simulink model "highwind"  (Simulink 8.0)
settings: Solver=ode45  StartTime=0.0  StopTime=300.0  RelTol=1e-3
undefined symbols (not defined in the file or in its folder): c1, c2, c3, c4, c5, c6, ctrlpara, Jg, Jr, K, Kt, R, ro_air, xishu
libraries: simulink_need_slupdate x1, wt_blockset_v3 x1
settings Model: Creator=acer  LastModifiedBy=Administrator
settings DataIOCC: SignalLoggingSaveFormat=ModelDataLogs
settings DebuggingCC: FcnCallInpInsideContextMsg=UseLocalSettings  StrictBusMsg=Warning
settings GRTTargetCC: CombineOutputUpdateFcns=off  GRTInterface=on

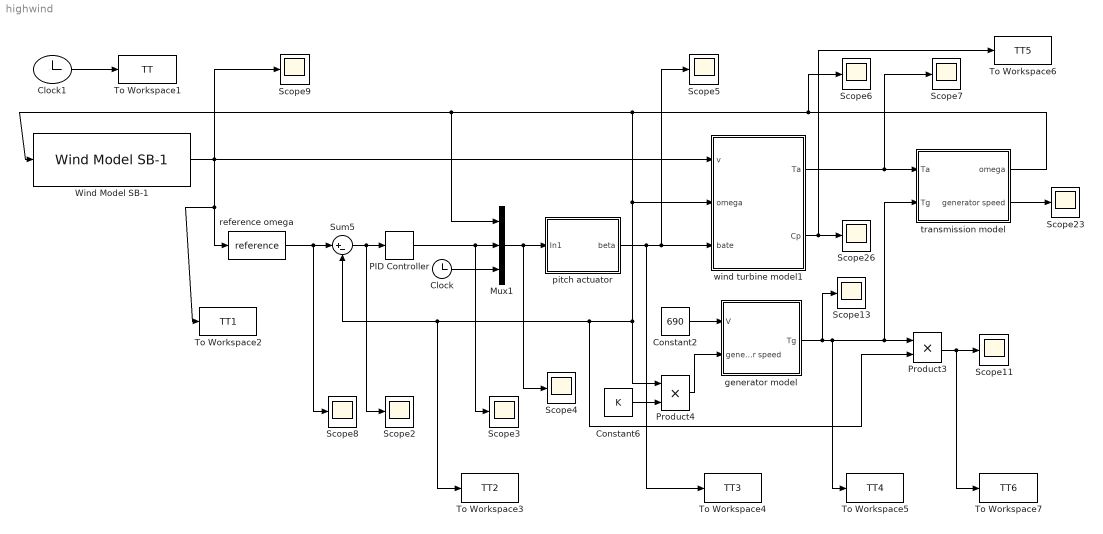
== system highwind ==
  Clock : Clock
  Clock1 : Clock
  Constant2 : Constant  Value=690
  Constant6 : Constant  Value=K
  Mux1 : Mux  Inputs=3
  PID Controller : simulink_need_slupdate/PID Controller  P=ctrlpara(1)  I=ctrlpara(2)  D=0
  Product3 : Product  RndMeth=Zero
  Product4 : Product  RndMeth=Zero
  Scope{2..9,11,13,23,26} (12 alike) : Scope
      Scope11 settings: TimeRange=100  YMin=1.455e+006  YMax=1.555e+006  SaveName=paper_goodoutput
      Scope13 settings: YMin=-35000  YMax=20000  SaveName=paper_goodTe
      Scope2 settings: TimeRange=100  YMin=-2e-005  YMax=2.25e-005  SaveName=paper_goodoutput1
      Scope23 settings: TimeRange=120  YMin=149.243  YMax=149.253
      Scope26 settings: YMin=-200000  YMax=350000  SaveName=ScopeData2
      Scope3 settings: TimeRange=100  YMin=-3250  YMax=1250  SaveName=paper_goodoutput2
      Scope4 settings: TimeRange=100  YMin=0  YMax=90  SaveName=paper_goodoutput3
      Scope5 settings: TimeRange=100  YMin=25.25  YMax=29.25  SaveName=paper_goodoutput4
      Scope6 settings: TimeRange=100  YMin=1.96995  YMax=1.97005  SaveName=paper_goodoutput5
      Scope7 settings: TimeRange=100  YMin=1.3475e+006  YMax=1.38e+006  SaveName=paper_goodoutput6
      Scope8 settings: TimeRange=100  YMin=1.9  YMax=2.1  SaveName=paper_goodoutput7
      Scope9 settings: TimeRange=100  YMin=16.65  YMax=17.6  SaveName=paper_goodoutput8
  Sum5 : Sum  Inputs=|+-  SaturateOnIntegerOverflow=on
  To Workspace1 : ToWorkspace  VariableName=TT  SampleTime=-1
  To Workspace2 : ToWorkspace  VariableName=TT1  SampleTime=-1
  To Workspace3 : ToWorkspace  VariableName=TT2  SampleTime=-1
  To Workspace4 : ToWorkspace  VariableName=TT3  SampleTime=-1
  To Workspace5 : ToWorkspace  VariableName=TT4  SampleTime=-1
  To Workspace6 : ToWorkspace  VariableName=TT5  SampleTime=-1
  To Workspace7 : ToWorkspace  VariableName=TT6  SampleTime=-1
  Wind Model SB-1 : wt_blockset_v3/Mechanical Components/Wind Model SB-1  D_rotor=72  v_mean=18  roughness=100  turb_int=12  T_sample=1
  generator model : Subsystem
  pitch actuator : Subsystem
  reference omega : MATLABFcn  MATLABFcn=reference
  transmission model : Subsystem
  wind turbine model1 : Subsystem
  wires:
  PID Controller/1 -> Mux1/2, Scope3/1
  Clock/1 -> Mux1/3
  transmission model/2(generator speed) -> Scope23/1
  Constant2/1 -> generator model/1(V)
  transmission model/1(omega) -> wind turbine model1/2(omega), Product4/1, Sum5/2, To Workspace3/1, Product3/2, Mux1/1, Wind Model SB-1/1, Scope6/1
  Product3/1 -> Scope11/1, To Workspace7/1
  wind turbine model1/2(Cp) -> Scope26/1, To Workspace6/1
  Constant6/1 -> Product4/2
  Product4/1 -> generator model/2(generator speed)
  wind turbine model1/1(Ta) -> transmission model/1(Ta), Scope7/1
  Sum5/1 -> PID Controller/1, Scope2/1
  Wind Model SB-1/1 -> wind turbine model1/1(v), Scope9/1, reference omega/1, To Workspace2/1
  pitch actuator/1(beta) -> wind turbine model1/3(bate), Scope5/1, To Workspace4/1
  Mux1/1 -> pitch actuator/1(In1), Scope4/1
  reference omega/1 -> Sum5/1, Scope8/1
  Clock1/1 -> To Workspace1/1
  generator model/1(Tg) -> Product3/1, transmission model/2(Tg), To Workspace5/1, Scope13/1

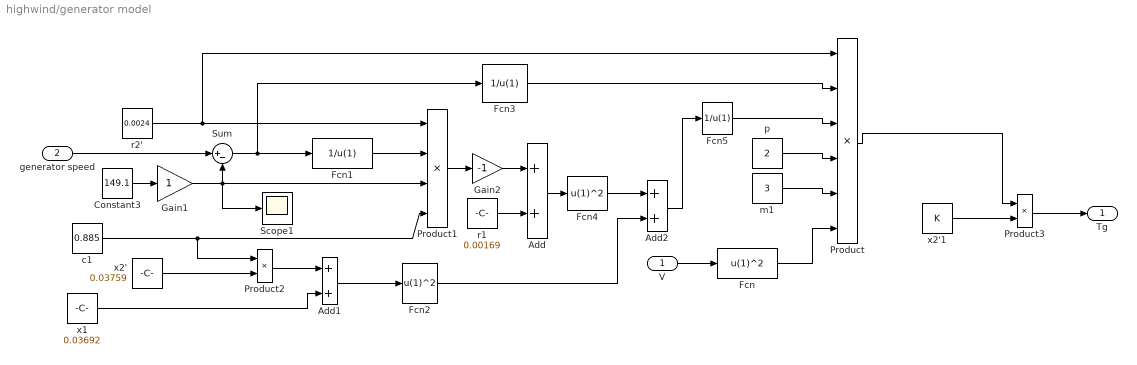
== system highwind/generator model ==
  V : Inport
  generator speed : Inport  Port=2
  Add : Sum
  Add1 : Sum
  Add2 : Sum
  Constant3 : Constant  Value=149.1
  Fcn : Fcn  Expr=u(1)^2
  Fcn1 : Fcn  Expr=1/u(1)
  Fcn2 : Fcn  Expr=u(1)^2
  Fcn3 : Fcn  Expr=1/u(1)
  Fcn4 : Fcn  Expr=u(1)^2
  Fcn5 : Fcn  Expr=1/u(1)
  Gain1 : Gain
  Gain2 : Gain  Gain=-1
  Product : Product  Inputs=6  RndMeth=Zero
  Product1 : Product  Inputs=4  RndMeth=Zero
  Product2 : Product  RndMeth=Zero
  Product3 : Product  RndMeth=Zero
  Scope1 : Scope
      settings: SaveName=ScopeData10
  Sum : Sum  Inputs=|+-
  c1 : Constant  Value=0.885
  m1 : Constant  Value=3
  p : Constant  Value=2
  r1 : Constant  Value=0.00169
  r2' : Constant  Value=0.0024
  x1 : Constant  Value=0.03692
  x2' : Constant  Value=0.03759
  x2'1 : Constant  Value=K
  Tg : Outport
  wires:
  V/1 -> Fcn/1
  generator speed/1 -> Sum/1
  Constant3/1 -> Gain1/1
  Gain1/1 -> Sum/2, Product1/3, Scope1/1
  Sum/1 -> Fcn3/1, Fcn1/1
  r2'/1 -> Product1/1, Product/1
  Fcn1/1 -> Product1/2
  c1/1 -> Product1/4, Product2/1
  x2'/1 -> Product2/2
  Product2/1 -> Add1/1
  x1/1 -> Add1/2
  Add1/1 -> Fcn2/1
  Product1/1 -> Gain2/1
  r1/1 -> Add/2
  Gain2/1 -> Add/1
  Add/1 -> Fcn4/1
  Fcn4/1 -> Add2/1
  Fcn2/1 -> Add2/2
  Add2/1 -> Fcn5/1
  Product/1 -> Product3/1
  Fcn3/1 -> Product/2
  Fcn5/1 -> Product/3
  p/1 -> Product/4
  m1/1 -> Product/5
  Fcn/1 -> Product/6
  x2'1/1 -> Product3/2
  Product3/1 -> Tg/1

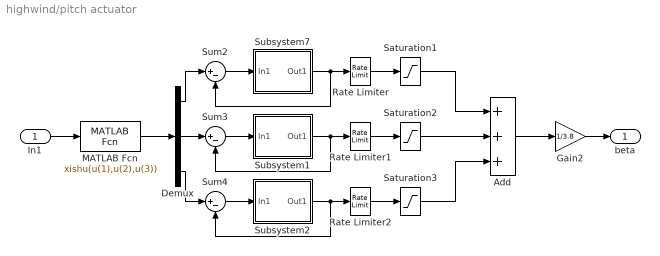
== system highwind/pitch actuator ==
  In1 : Inport
  Add : Sum  Inputs=+++
  Demux : Demux  Outputs=3
  Gain2 : Gain  Gain=1/3.8
  MATLAB Fcn : MATLABFcn  MATLABFcn=xishu(u(1),u(2),u(3))
  Rate Limiter : RateLimiter  RisingSlewLimit=5  FallingSlewLimit=-5
  Rate Limiter1 : RateLimiter  RisingSlewLimit=5  FallingSlewLimit=-5
  Rate Limiter2 : RateLimiter  RisingSlewLimit=5  FallingSlewLimit=-5
  Saturation1 : Saturate  UpperLimit=90  LowerLimit=-90
  Saturation2 : Saturate  UpperLimit=90  LowerLimit=-90
  Saturation3 : Saturate  UpperLimit=90  LowerLimit=-90
  Subsystem1 : Subsystem
  Subsystem2 : Subsystem
  Subsystem7 : Subsystem
  Sum2 : Sum  Inputs=|+-  SaturateOnIntegerOverflow=on
  Sum3 : Sum  Inputs=|+-  SaturateOnIntegerOverflow=on
  Sum4 : Sum  Inputs=|+-  SaturateOnIntegerOverflow=on
  beta : Outport
  wires:
  Subsystem7/1(Out1) -> Sum2/2, Rate Limiter/1
  Sum2/1 -> Subsystem7/1(In1)
  Subsystem1/1(Out1) -> Sum3/2, Rate Limiter1/1
  Sum3/1 -> Subsystem1/1(In1)
  MATLAB Fcn/1 -> Demux/1
  Demux/2 -> Sum3/1
  Demux/1 -> Sum2/1
  Demux/3 -> Sum4/1
  Saturation1/1 -> Add/1
  Add/1 -> Gain2/1
  Gain2/1 -> beta/1
  In1/1 -> MATLAB Fcn/1
  Rate Limiter/1 -> Saturation1/1
  Rate Limiter1/1 -> Saturation2/1
  Rate Limiter2/1 -> Saturation3/1
  Saturation2/1 -> Add/2
  Saturation3/1 -> Add/3
  Subsystem2/1(Out1) -> Rate Limiter2/1, Sum4/2
  Sum4/1 -> Subsystem2/1(In1)

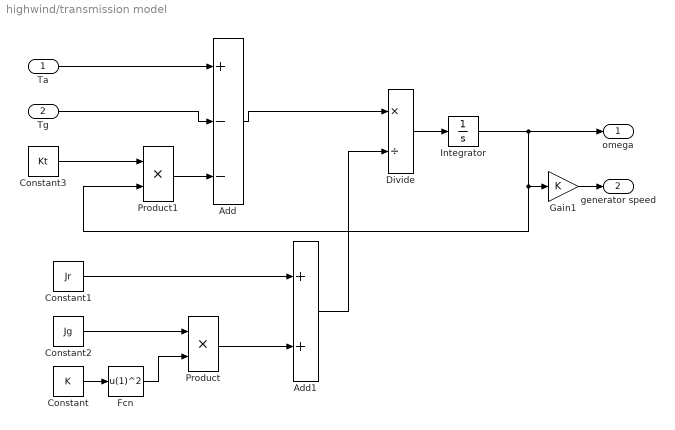
== system highwind/transmission model ==
  Ta : Inport
  Tg : Inport  Port=2
  Add : Sum  Inputs=+--
  Add1 : Sum
  Constant : Constant  Value=K
  Constant1 : Constant  Value=Jr
  Constant2 : Constant  Value=Jg
  Constant3 : Constant  Value=Kt  VectorParams1D=off
  Divide : Product  Inputs=*/
  Fcn : Fcn  Expr=u(1)^2
  Gain1 : Gain  Gain=K
  Integrator : Integrator  InitialCondition=1.96885526
  Product : Product  RndMeth=Zero
  Product1 : Product  RndMeth=Zero
  omega : Outport
  generator speed : Outport  Port=2
  wires:
  Fcn/1 -> Product/2
  Constant/1 -> Fcn/1
  Tg/1 -> Add/2
  Ta/1 -> Add/1
  Constant2/1 -> Product/1
  Constant1/1 -> Add1/1
  Product/1 -> Add1/2
  Add/1 -> Divide/1
  Add1/1 -> Divide/2
  Divide/1 -> Integrator/1
  Integrator/1 -> omega/1, Gain1/1, Product1/2
  Gain1/1 -> generator speed/1
  Product1/1 -> Add/3
  Constant3/1 -> Product1/1

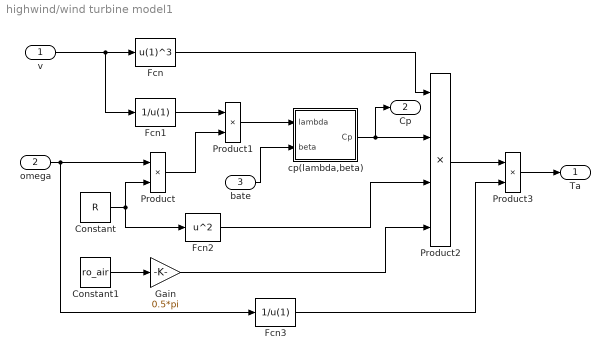
== system highwind/wind turbine model1 ==
  v : Inport
  omega : Inport  Port=2
  bate : Inport  Port=3
  Constant : Constant  Value=R
  Constant1 : Constant  Value=ro_air
  Fcn : Fcn  Expr=u(1)^3
  Fcn1 : Fcn  Expr=1/u(1)
  Fcn2 : Fcn  Expr=u^2
  Fcn3 : Fcn  Expr=1/u(1)
  Gain : Gain  Gain=0.5*pi
  Product : Product  RndMeth=Zero
  Product1 : Product  RndMeth=Zero
  Product2 : Product  Inputs=4  RndMeth=Zero
  Product3 : Product  RndMeth=Zero
  cp(lambda,beta) : Subsystem  AncestorBlock=DRlib/Wind Generation/Wind Turbine/cp(lambda,beta)
  Ta : Outport
  Cp : Outport  Port=2
  wires:
  v/1 -> Fcn/1, Fcn1/1
  omega/1 -> Product/1, Fcn3/1
  Constant/1 -> Product/2, Fcn2/1
  Fcn1/1 -> Product1/1
  Product/1 -> Product1/2
  Product1/1 -> cp(lambda,beta)/1(lambda)
  bate/1 -> cp(lambda,beta)/2(beta)
  Fcn/1 -> Product2/1
  cp(lambda,beta)/1(Cp) -> Product2/2, Cp/1
  Fcn2/1 -> Product2/3
  Gain/1 -> Product2/4
  Constant1/1 -> Gain/1
  Product2/1 -> Product3/1
  Fcn3/1 -> Product3/2
  Product3/1 -> Ta/1

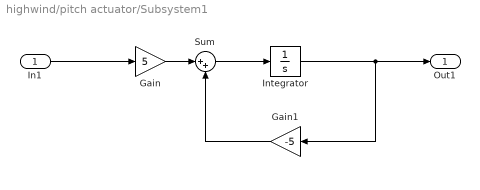
== system highwind/pitch actuator/Subsystem1 ==
  In1 : Inport
  Gain : Gain  Gain=5
  Gain1 : Gain  Gain=-5
  Integrator : Integrator  InitialCondition=25
  Sum : Sum  Inputs=|++
  Out1 : Outport
  wires:
  Integrator/1 -> Gain1/1, Out1/1
  Gain1/1 -> Sum/2
  Sum/1 -> Integrator/1
  Gain/1 -> Sum/1
  In1/1 -> Gain/1

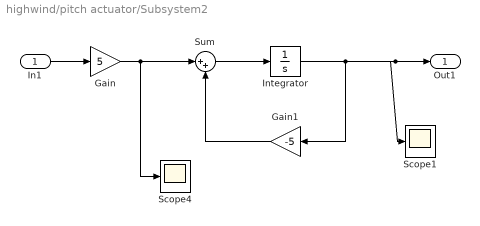
== system highwind/pitch actuator/Subsystem2 ==
  In1 : Inport
  Gain : Gain  Gain=5
  Gain1 : Gain  Gain=-5
  Integrator : Integrator  InitialCondition=25
  Scope1 : Scope
      settings: YMin=-1.2e+019  YMax=1e+018  SaveName=ScopeData19
  Scope4 : Scope
      settings: TimeRange=40  YMin=-6.475243243197446e+026  YMax=-2.489945945900152e+026  SaveName=ScopeData18
  Sum : Sum  Inputs=|++
  Out1 : Outport
  wires:
  Integrator/1 -> Gain1/1, Out1/1, Scope1/1
  Gain1/1 -> Sum/2
  Sum/1 -> Integrator/1
  Gain/1 -> Sum/1, Scope4/1
  In1/1 -> Gain/1

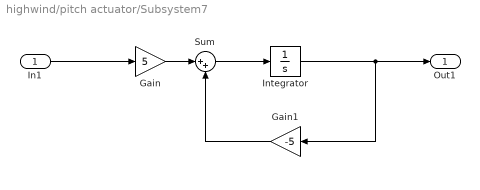
== system highwind/pitch actuator/Subsystem7 ==
  In1 : Inport
  Gain : Gain  Gain=5
  Gain1 : Gain  Gain=-5
  Integrator : Integrator  InitialCondition=25
  Sum : Sum  Inputs=|++
  Out1 : Outport
  wires:
  Integrator/1 -> Gain1/1, Out1/1
  Gain1/1 -> Sum/2
  Sum/1 -> Integrator/1
  Gain/1 -> Sum/1
  In1/1 -> Gain/1

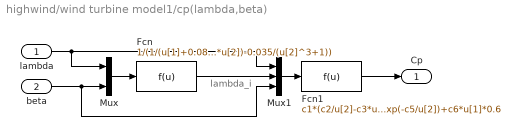
== system highwind/wind turbine model1/cp(lambda,beta) ==
  note: lambda_i
  lambda : Inport
  beta : Inport  Port=2
  Fcn : Fcn  Expr=1/(1/(u[1]+0.08*u[2])-0.035/(u[2]^3+1))
  Fcn1 : Fcn  Expr=c1*(c2/u[2]-c3*u[3]-c4)*exp(-c5/u[2])+c6*u[1]*0.6
  Mux : Mux  Inputs=2
  Mux1 : Mux  Inputs=3
  Cp : Outport
  wires:
  Fcn/1 -> Mux1/2
  Fcn1/1 -> Cp/1
  lambda/1 -> Mux1/1, Mux/1
  Mux1/1 -> Fcn1/1
  beta/1 -> Mux1/3, Mux/2
  Mux/1 -> Fcn/1
